simulink subsystem "integrador_trapecios"  (R2023b)
settings: Solver=VariableStepAuto  StartTime=0.0  StopTime=10.0  RelTol=1e-3
values from neighbouring files (symbols this model uses):
  Ts = 2*pi/(10*5000)    (= 0.000125663706144)    [constantes.m]    (also in test_polos_PID.m = 40)
settings Model: Creator=rodri  LastModifiedBy=Nahuel

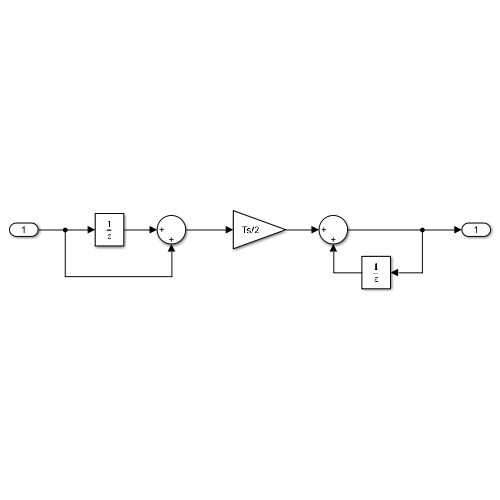
[thumbnail: Simulink's stored preview of the top-level diagram]
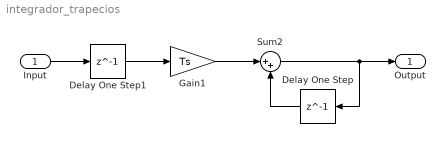
== system integrador_trapecios ==
  Input : Inport
  Delay One Step : Delay  DelayLength=1
  Delay One Step1 : Delay  DelayLength=1
  Gain1 : Gain  Gain=Ts
  Sum2 : Sum  Inputs=|++
  Output : Outport
  wires:
  Delay One Step/1 -> Sum2/2
  Sum2/1 -> Delay One Step/1, Output/1
  Delay One Step1/1 -> Gain1/1
  Input/1 -> Delay One Step1/1
  Gain1/1 -> Sum2/1
